simulink model "TrimControlSystemDesigner"  (R2024b)
settings: Solver=VariableStepAuto  StartTime=0.0  StopTime=10.0  RelTol=1e-3
values from neighbouring files (symbols this model uses):
  u1max = 25*pi/180    (= 0.436332312999)    [RCAM_model.m]
  u1min = -25*pi/180    (= -0.436332312999)    [RCAM_model.m]
  u2max = 10*pi/180    (= 0.174532925199)    [RCAM_model.m]
  u2min = -25*pi/180    (= -0.436332312999)    [RCAM_model.m]
  u3max = 30*pi/180    (= 0.523598775598)    [RCAM_model.m]
  u3min = - 30*pi/180    (= -0.523598775598)    [RCAM_model.m]
  u4max = 10*pi/180    (= 0.174532925199)    [RCAM_model.m]
  u5max = 10*pi/180    (= 0.174532925199)    [RCAM_model.m]
  u5min = 0.5*pi/180    (= 0.00872664625997)    [RCAM_model.m]
  x0 = [85 ... (first row only)    [sim_initialise.m]
undefined symbols (not defined in the file or in its folder): RCAM_model_new, u14min
settings Model: Creator=satvik_sh  LastModifiedBy=satvik_sh

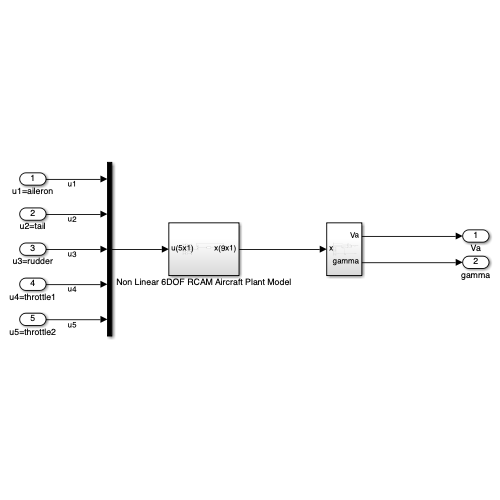
[thumbnail: Simulink's stored preview of the top-level diagram]
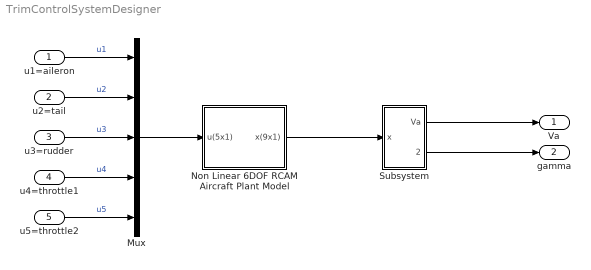
== system TrimControlSystemDesigner ==
  u1=aileron : Inport
  u2=tail : Inport  Port=2
  u3=rudder : Inport  Port=3
  u4=throttle1 : Inport  Port=4
  u5=throttle2 : Inport  Port=5
  Mux : Mux  Inputs=5
  Non Linear 6DOF RCAM Aircraft Plant Model : Subsystem
  Subsystem : Subsystem
  Va : Outport
  gamma : Outport  Port=2
  wires:
  u3=rudder/1 -> Mux/3  "u3"
  u4=throttle1/1 -> Mux/4  "u4"
  u5=throttle2/1 -> Mux/5  "u5"
  u2=tail/1 -> Mux/2  "u2"
  u1=aileron/1 -> Mux/1  "u1"
  Mux/1 -> Non Linear 6DOF RCAM Aircraft Plant Model/1(u(5x1))
  Subsystem/1(Va) -> Va/1
  Subsystem/2(gamma) -> gamma/1
  Non Linear 6DOF RCAM Aircraft Plant Model/1(x(9x1)) -> Subsystem/1(x)

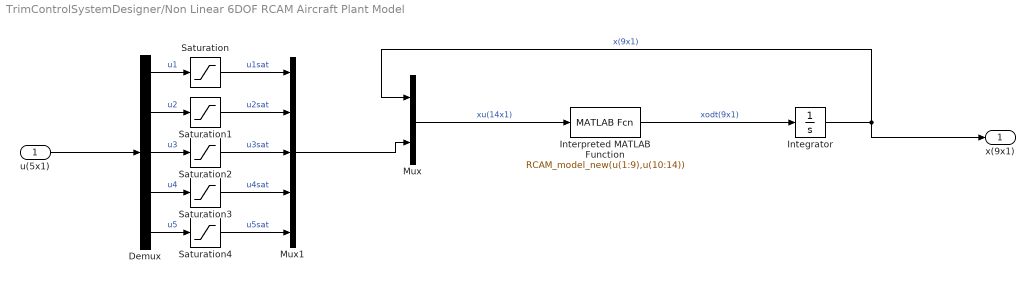
== system TrimControlSystemDesigner/Non Linear 6DOF RCAM Aircraft Plant Model ==
  u(5x1) : Inport
  Demux : Demux  Outputs=5
  Integrator : Integrator  InitialCondition=x0
  Interpreted MATLAB Function : MATLABFcn  MATLABFcn=RCAM_model_new(u(1:9),u(10:14))
  Mux : Mux  Inputs=2
  Mux1 : Mux  Inputs=5
  Saturation : Saturate  UpperLimit=u1max  LowerLimit=u1min
  Saturation1 : Saturate  UpperLimit=u2max  LowerLimit=u2min
  Saturation2 : Saturate  UpperLimit=u3max  LowerLimit=u3min
  Saturation3 : Saturate  UpperLimit=u4max  LowerLimit=u14min
  Saturation4 : Saturate  UpperLimit=u5max  LowerLimit=u5min
  x(9x1) : Outport
  wires:
  Interpreted MATLAB Function/1 -> Integrator/1  "xodt(9x1)"
  Mux/1 -> Interpreted MATLAB Function/1  "xu(14x1)"
  Integrator/1 -> x(9x1)/1, Mux/1  "x(9x1)"
  u(5x1)/1 -> Demux/1
  Demux/1 -> Saturation/1  "u1"
  Demux/2 -> Saturation1/1  "u2"
  Demux/3 -> Saturation2/1  "u3"
  Demux/4 -> Saturation3/1  "u4"
  Demux/5 -> Saturation4/1  "u5"
  Saturation/1 -> Mux1/1  "u1sat"
  Saturation1/1 -> Mux1/2  "u2sat"
  Saturation2/1 -> Mux1/3  "u3sat"
  Saturation3/1 -> Mux1/4  "u4sat"
  Saturation4/1 -> Mux1/5  "u5sat"
  Mux1/1 -> Mux/2

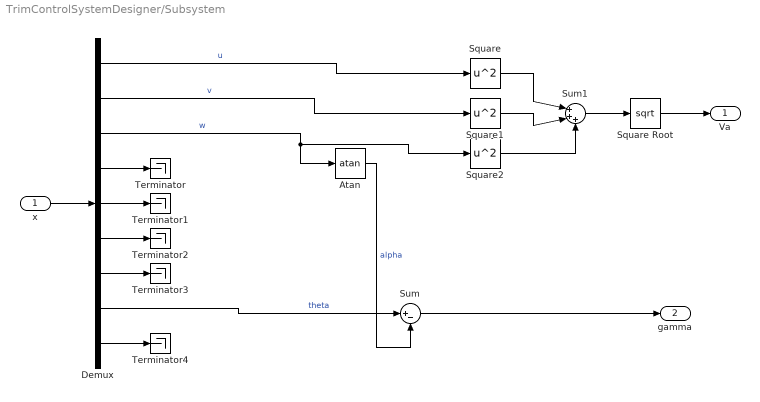
== system TrimControlSystemDesigner/Subsystem ==
  x : Inport
  Atan : Trigonometry  Operator=atan
  Demux : Demux  Outputs=9
  Square : Math  Operator=square
  Square Root : Sqrt
  Square1 : Math  Operator=square
  Square2 : Math  Operator=square
  Sum : Sum  Inputs=|+-
  Sum1 : Sum  Inputs=|+++
  Terminator{,1..4} (5 alike) : Terminator
  Va : Outport
  gamma : Outport  Port=2
  wires:
  Sum1/1 -> Square Root/1
  Demux/2 -> Square1/1  "v"
  Square1/1 -> Sum1/2
  Square Root/1 -> Va/1
  Sum/1 -> gamma/1
  Demux/4 -> Terminator/1
  Demux/5 -> Terminator1/1
  Demux/7 -> Terminator3/1
  Square/1 -> Sum1/1
  Square2/1 -> Sum1/3
  Demux/6 -> Terminator2/1
  x/1 -> Demux/1
  Demux/3 -> Atan/1, Square2/1  "w"
  Atan/1 -> Sum/2  "alpha"
  Demux/1 -> Square/1  "u"
  Demux/8 -> Sum/1  "theta"
  Demux/9 -> Terminator4/1
